simulink model "ekf1"  (R2023b)
settings: Solver=FixedStepAuto  StartTime=0.0  StopTime=Tend_slk  FixedStep=Ts_slk  RelTol=1e-3
values from neighbouring files (symbols this model uses):
  IMU_w_b_bias = IMU_var_bias_matrix(:,2)    [ekf1_script.m]    (also in ekf2_script.m; ekf3_script.m)
  meas_pole = 15    [ekf1_script.m]    (also in ekf2_script.m = 3; ekf3_script.m)
  P0 = diag([P0_ph,P0_th,P0_ps,P0_bias_wp,P0_bias_wq,P0_bias_wr])    [ekf1_script.m]
  Q = diag([q_ph,q_th,q_ps,q_bias_w_b,q_bias_w_b,q_bias_w_b])    [ekf1_script.m]
  R = diag([r_th,r_th,r_ps])    [ekf1_script.m]
  Ts_EKF_integr = 0.001    [complementary_filter_script.m]    (also in ekf1_script.m = 0.0001; ekf2_script.m = 0.0001; ekf3_script.m = 0.0001)
  Ts_EKF_meas = 0.01    [complementary_filter_script.m]    (also in ekf1_script.m; ekf2_script.m; ekf3_script.m)
  Ts_slk = 0.01    [complementary_filter_script.m]    (also in ekf1_script.m; ekf2_script.m; ekf3_script.m)
  x0EKF = [ph0;th0;ps0;bias_wp0;bias_wq0;bias_wr0]    [ekf1_script.m]
settings Model: Creator=teoma  LastModifiedBy=teoma

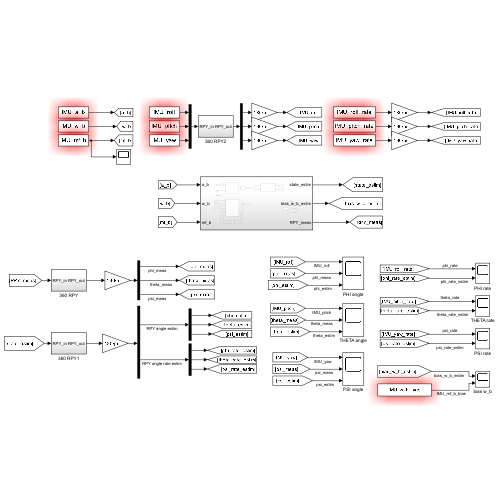
[thumbnail: Simulink's stored preview of the top-level diagram]
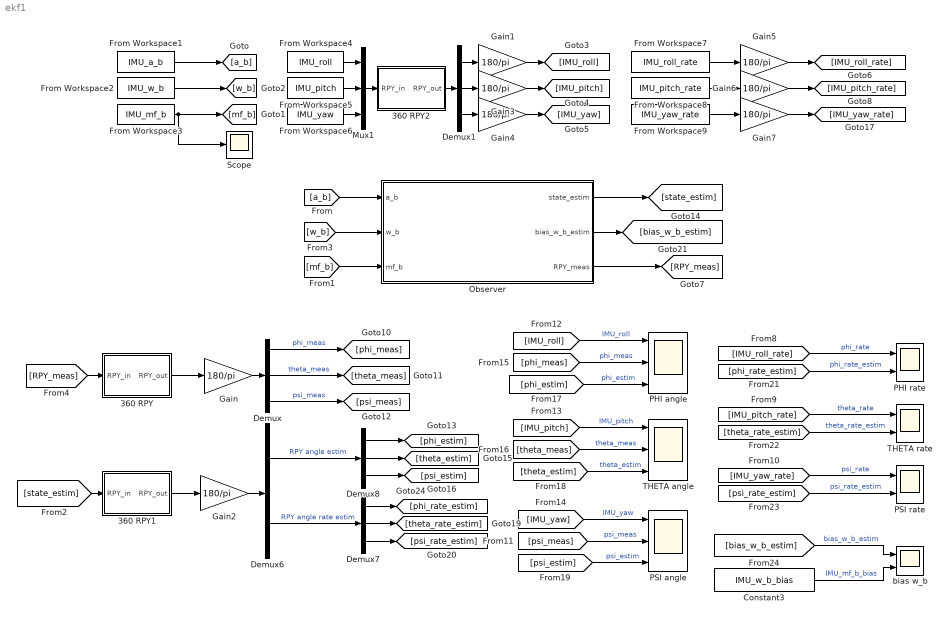
== system ekf1 ==
  360 RPY : Subsystem
  360 RPY1 : Subsystem
  360 RPY2 : Subsystem
  Constant3 : Constant  Value=IMU_w_b_bias
  Demux{,1,7..8} (4 alike) : Demux  Outputs=3
  Demux6 : Demux  Outputs=2
  From Workspace1 : FromWorkspace  VariableName=IMU_a_b  OutDataTypeStr=double  SampleTime=Ts_slk  Interpolate=off  OutputAfterFinalValue=Setting to zero
  From Workspace2 : FromWorkspace  VariableName=IMU_w_b  OutDataTypeStr=double  SampleTime=Ts_slk  Interpolate=off  OutputAfterFinalValue=Setting to zero
  From Workspace3 : FromWorkspace  VariableName=IMU_mf_b  OutDataTypeStr=double  SampleTime=Ts_slk  Interpolate=off  OutputAfterFinalValue=Setting to zero
  From Workspace4 : FromWorkspace  VariableName=IMU_roll  OutDataTypeStr=double  SampleTime=Ts_slk  Interpolate=off  OutputAfterFinalValue=Setting to zero
  From Workspace5 : FromWorkspace  VariableName=IMU_pitch  OutDataTypeStr=double  SampleTime=Ts_slk  Interpolate=off  OutputAfterFinalValue=Setting to zero
  From Workspace6 : FromWorkspace  VariableName=IMU_yaw  OutDataTypeStr=double  SampleTime=Ts_slk  Interpolate=off  OutputAfterFinalValue=Setting to zero
  From Workspace7 : FromWorkspace  VariableName=IMU_roll_rate  OutDataTypeStr=double  SampleTime=Ts_slk  Interpolate=off  OutputAfterFinalValue=Setting to zero
  From Workspace8 : FromWorkspace  VariableName=IMU_pitch_rate  OutDataTypeStr=double  SampleTime=Ts_slk  Interpolate=off  OutputAfterFinalValue=Setting to zero
  From Workspace9 : FromWorkspace  VariableName=IMU_yaw_rate  OutDataTypeStr=double  SampleTime=Ts_slk  Interpolate=off  OutputAfterFinalValue=Setting to zero
  Gain{,1..7} (8 alike) : Gain  Gain=180/pi
  Mux1 : Mux  Inputs=3
  Observer : Subsystem
  PHI angle : Scope  NumInputPorts=3
  PHI rate : Scope  NumInputPorts=2
  PSI angle : Scope  NumInputPorts=3
  PSI rate : Scope  NumInputPorts=2
  Scope : Scope
  THETA angle : Scope  NumInputPorts=3
  THETA rate : Scope  NumInputPorts=2
  bias w_b : Scope  NumInputPorts=2
  wires:
  Constant3/1 -> bias w_b/2  "IMU_mf_b_bias"
  [bias_w_b_estim] -> bias w_b/1  "bias_w_b_estim"
  [IMU_yaw_rate] -> PSI rate/1  "psi_rate"
  [theta_estim] -> THETA angle/3  "theta_estim"
  [theta_rate_estim] -> THETA rate/2  "theta_rate_estim"
  [IMU_pitch_rate] -> THETA rate/1  "theta_rate"
  [IMU_roll_rate] -> PHI rate/1  "phi_rate"
  [phi_rate_estim] -> PHI rate/2  "phi_rate_estim"
  [phi_estim] -> PHI angle/3  "phi_estim"
  [psi_estim] -> PSI angle/3  "psi_estim"
  [theta_meas] -> THETA angle/2  "theta_meas"
  [IMU_yaw] -> PSI angle/1  "IMU_yaw"
  [phi_meas] -> PHI angle/2  "phi_meas"
  [IMU_pitch] -> THETA angle/1  "IMU_pitch"
  [psi_rate_estim] -> PSI rate/2  "psi_rate_estim"
  [psi_meas] -> PSI angle/2  "psi_meas"
  [IMU_roll] -> PHI angle/1  "IMU_roll"
  From Workspace1/1 -> [a_b]
  From Workspace2/1 -> [w_b]
  From Workspace9/1 -> Gain7/1
  From Workspace8/1 -> Gain6/1
  From Workspace7/1 -> Gain5/1
  Gain5/1 -> [IMU_roll_rate]
  Gain6/1 -> [IMU_pitch_rate]
  Gain7/1 -> [IMU_yaw_rate]
  From Workspace3/1 -> [mf_b], Scope/1
  [mf_b] -> Observer/3(mf_b)
  [a_b] -> Observer/1(a_b)
  Observer/1(state_estim) -> [state_estim]
  Observer/2(bias_w_b_estim) -> [bias_w_b_estim]
  Observer/3(RPY_meas) -> [RPY_meas]
  [w_b] -> Observer/2(w_b)
  Demux8/2 -> [theta_estim]
  Demux8/3 -> [psi_estim]
  Demux7/3 -> [psi_rate_estim]
  Demux/2 -> [theta_meas]  "theta_meas"
  Gain/1 -> Demux/1
  Demux6/2 -> Demux7/1  "RPY angle rate estim"
  Demux7/2 -> [theta_rate_estim]
  360 RPY1/1(RPY_out) -> Gain2/1
  Demux6/1 -> Demux8/1  "RPY angle estim"
  360 RPY/1(RPY_out) -> Gain/1
  Demux8/1 -> [phi_estim]
  Demux7/1 -> [phi_rate_estim]
  Demux/3 -> [psi_meas]  "psi_meas"
  Gain2/1 -> Demux6/1
  Demux/1 -> [phi_meas]  "phi_meas"
  [state_estim] -> 360 RPY1/1(RPY_in)
  [RPY_meas] -> 360 RPY/1(RPY_in)
  Mux1/1 -> 360 RPY2/1(RPY_in)
  Demux1/1 -> Gain1/1
  From Workspace4/1 -> Mux1/1
  Gain1/1 -> [IMU_roll]
  Gain3/1 -> [IMU_pitch]
  Demux1/2 -> Gain3/1
  Demux1/3 -> Gain4/1
  From Workspace5/1 -> Mux1/2
  Gain4/1 -> [IMU_yaw]
  From Workspace6/1 -> Mux1/3
  360 RPY2/1(RPY_out) -> Demux1/1

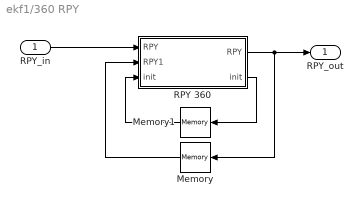
== system ekf1/360 RPY ==
  RPY_in : Inport
  Memory : Memory
  Memory1 : Memory
  RPY 360 : MATLAB Function  TreatAsAtomicUnit=on
  RPY_out : Outport
  wires:
  Memory/1 -> RPY 360/2(RPY1)
  Memory1/1 -> RPY 360/3("init ")
  RPY 360/2(init) -> Memory1/1
  RPY 360/1(RPY) -> Memory/1, RPY_out/1
  RPY_in/1 -> RPY 360/1("RPY ")

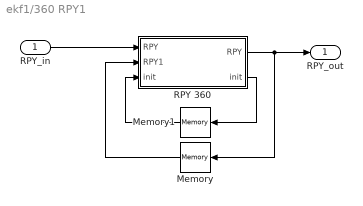
== system ekf1/360 RPY1 ==
  RPY_in : Inport
  Memory : Memory
  Memory1 : Memory
  RPY 360 : MATLAB Function  TreatAsAtomicUnit=on
  RPY_out : Outport
  wires:
  Memory/1 -> RPY 360/2(RPY1)
  Memory1/1 -> RPY 360/3("init ")
  RPY 360/2(init) -> Memory1/1
  RPY 360/1(RPY) -> Memory/1, RPY_out/1
  RPY_in/1 -> RPY 360/1("RPY ")

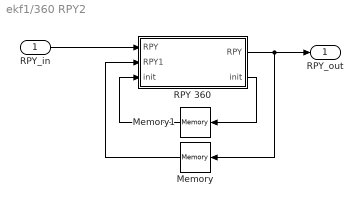
== system ekf1/360 RPY2 ==
  RPY_in : Inport
  Memory : Memory
  Memory1 : Memory
  RPY 360 : MATLAB Function  TreatAsAtomicUnit=on
  RPY_out : Outport
  wires:
  RPY_in/1 -> RPY 360/1("RPY ")
  RPY 360/1(RPY) -> Memory/1, RPY_out/1
  Memory/1 -> RPY 360/2(RPY1)
  RPY 360/2(init) -> Memory1/1
  Memory1/1 -> RPY 360/3("init ")

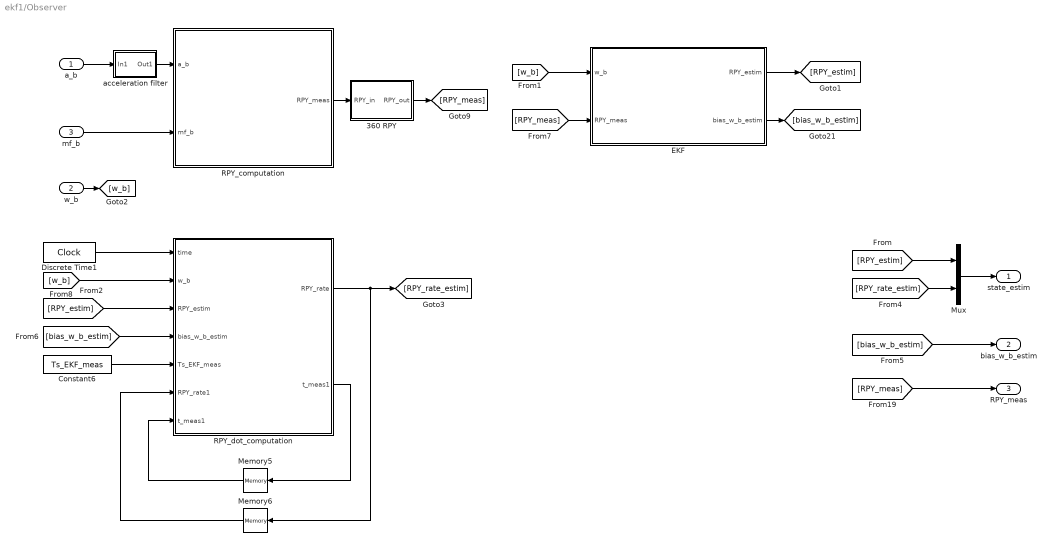
== system ekf1/Observer ==
  a_b : Inport
  w_b : Inport  Port=2
  mf_b : Inport  Port=3
  360 RPY : Subsystem
  Constant6 : Constant  Value=Ts_EKF_meas
  Discrete Time1 : DigitalClock  SampleTime=Ts_slk
  EKF : Subsystem
  Memory5 : Memory
  Memory6 : Memory
  Mux : Mux  Inputs=2
  RPY_computation : MATLAB Function  TreatAsAtomicUnit=on
  RPY_dot_computation : MATLAB Function  TreatAsAtomicUnit=on
  acceleration filter : Subsystem  mask{p=meas_pole}
      mask prompts: p "pole (p)"
  state_estim : Outport
  bias_w_b_estim : Outport  Port=2
  RPY_meas : Outport  Port=3
  wires:
  [w_b] -> EKF/1(w_b)
  EKF/1(RPY_estim) -> [RPY_estim]
  a_b/1 -> acceleration filter/1(In1)
  acceleration filter/1(Out1) -> RPY_computation/1(a_b)
  [RPY_meas] -> EKF/2(RPY_meas)
  EKF/2(bias_w_b_estim) -> [bias_w_b_estim]
  RPY_computation/1(RPY_meas) -> 360 RPY/1(RPY_in)
  mf_b/1 -> RPY_computation/2(mf_b)
  Memory5/1 -> RPY_dot_computation/7("t_meas1 ")
  Discrete Time1/1 -> RPY_dot_computation/1(time)
  RPY_dot_computation/2(t_meas1) -> Memory5/1
  [w_b] -> RPY_dot_computation/2(w_b)
  Memory6/1 -> RPY_dot_computation/6(RPY_rate1)
  RPY_dot_computation/1(RPY_rate) -> [RPY_rate_estim], Memory6/1
  Constant6/1 -> RPY_dot_computation/5(Ts_EKF_meas)
  [RPY_estim] -> RPY_dot_computation/3(RPY_estim)
  [bias_w_b_estim] -> RPY_dot_computation/4(bias_w_b_estim)
  w_b/1 -> [w_b]
  [RPY_meas] -> RPY_meas/1
  [bias_w_b_estim] -> bias_w_b_estim/1
  Mux/1 -> state_estim/1
  [RPY_estim] -> Mux/1
  [RPY_rate_estim] -> Mux/2
  360 RPY/1(RPY_out) -> [RPY_meas]

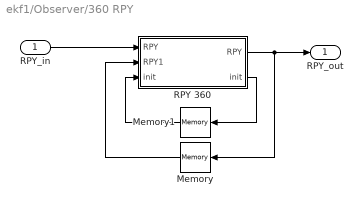
== system ekf1/Observer/360 RPY ==
  RPY_in : Inport
  Memory : Memory
  Memory1 : Memory
  RPY 360 : MATLAB Function  TreatAsAtomicUnit=on
  RPY_out : Outport
  wires:
  RPY_in/1 -> RPY 360/1("RPY ")
  RPY 360/1(RPY) -> Memory/1, RPY_out/1
  Memory/1 -> RPY 360/2(RPY1)
  RPY 360/2(init) -> Memory1/1
  Memory1/1 -> RPY 360/3("init ")

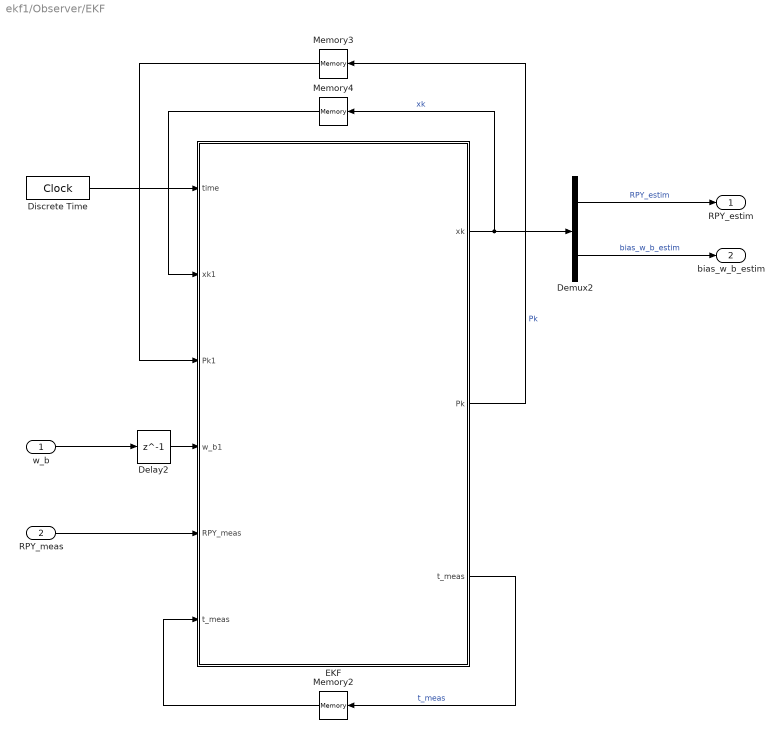
== system ekf1/Observer/EKF ==
  w_b : Inport
  RPY_meas : Inport  Port=2
  Delay2 : Delay  DelayLength=1  SampleTime=Ts_EKF_meas
  Demux2 : Demux  Outputs=2
  Discrete Time : DigitalClock  SampleTime=Ts_slk
  EKF : MATLAB Function  TreatAsAtomicUnit=on
  Memory2 : Memory
  Memory3 : Memory  InitialCondition=P0
  Memory4 : Memory  InitialCondition=x0EKF
  RPY_estim : Outport
  bias_w_b_estim : Outport  Port=2
  wires:
  w_b/1 -> Delay2/1
  EKF/2(Pk) -> Memory3/1  "Pk"
  Memory2/1 -> EKF/6("t_meas ")
  EKF/3(t_meas) -> Memory2/1  "t_meas"
  RPY_meas/1 -> EKF/5(RPY_meas)
  Discrete Time/1 -> EKF/1(time)
  Memory3/1 -> EKF/3(Pk1)
  Delay2/1 -> EKF/4(w_b1)
  Memory4/1 -> EKF/2(xk1)
  Demux2/2 -> bias_w_b_estim/1  "bias_w_b_estim"
  EKF/1(xk) -> Memory4/1, Demux2/1  "xk"
  Demux2/1 -> RPY_estim/1  "RPY_estim"

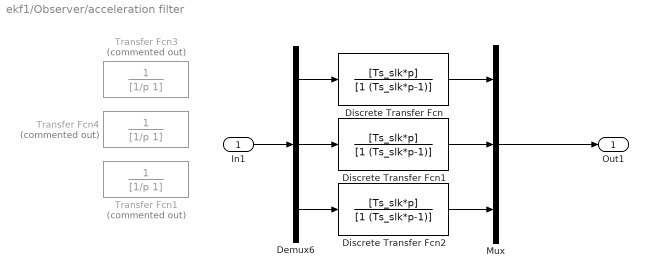
== system ekf1/Observer/acceleration filter ==
  In1 : Inport
  Demux6 : Demux  Outputs=3
  Discrete Transfer Fcn : DiscreteTransferFcn  Numerator=[Ts_slk*p]  Denominator=[1 (Ts_slk*p-1)]
  Discrete Transfer Fcn1 : DiscreteTransferFcn  Numerator=[Ts_slk*p]  Denominator=[1 (Ts_slk*p-1)]
  Discrete Transfer Fcn2 : DiscreteTransferFcn  Numerator=[Ts_slk*p]  Denominator=[1 (Ts_slk*p-1)]
  Mux : Mux  Inputs=3
  Transfer Fcn1 : TransferFcn  Commented=on  Denominator=[1/p 1]
  Transfer Fcn3 : TransferFcn  Commented=on  Denominator=[1/p 1]
  Transfer Fcn4 : TransferFcn  Commented=on  Denominator=[1/p 1]
  Out1 : Outport
  wires:
  Discrete Transfer Fcn1/1 -> Mux/2
  Demux6/3 -> Discrete Transfer Fcn2/1
  Mux/1 -> Out1/1
  Discrete Transfer Fcn2/1 -> Mux/3
  Discrete Transfer Fcn/1 -> Mux/1
  In1/1 -> Demux6/1
  Demux6/1 -> Discrete Transfer Fcn/1
  Demux6/2 -> Discrete Transfer Fcn1/1

== matlab function ekf1/Observer/RPY_dot_computation ==
  data: time input; w_b input; RPY_estim input; bias_w_b_estim input; Ts_EKF_meas input; RPY_rate1 input; RPY_rate output; t_meas1 input; t_meas1 output
function [RPY_rate,t_meas1] = RPY_dot_computation(time,w_b,RPY_estim,bias_w_b_estim,Ts_EKF_meas,RPY_rate1,t_meas1)

if time - t_meas1 >= Ts_EKF_meas || time == 0
    wp          =       w_b(1,1);               % p-dir of angular velocity w
    wq          =       w_b(2,1);               % q-dir of angular velocity w
    wr          =       w_b(3,1);               % r-dir of angular velocity w

    phi         =       RPY_estim(1,1);         % roll angle (rad)
    theta       =       RPY_estim(2,1);         % pitch angle (rad)
    psi         =       RPY_estim(3,1);         % yaw angle (rad)  
    bias_wp     =       bias_w_b_estim(1,1);    % bias of p-dir of angular velocity w
    bias_wq     =       bias_w_b_estim(2,1);    % bias of q-dir of angular velocity w
    bias_wr     =       bias_w_b_estim(3,1);   % bias of r-dir of angular velocity w

    cph         =       cos(phi);
    cth         =       cos(theta);
    cps         =       cos(psi);
    sph         =       sin(phi);
    sth         =       sin(theta);
    sps         =       sin(psi);
    tth         =       sth/cth;

    % integration step
    t_meas1 = time;
    W_eta = [1,    sph*tth,    cph*tth;
             0,    cph,        -sph;
             0,    sph/cth,    cph/cth;];
    w_b_corrected = [wp-bias_wp; wq-bias_wq; wr-bias_wr;];
    RPY_rate = W_eta*w_b_corrected;
else
    RPY_rate = RPY_rate1;
end
end

== matlab function ekf1/360 RPY1/RPY 360 ==
  data: RPY input; RPY output; RPY1 input; init output; init input
function [RPY,init] = RPY_360(RPY,RPY1,init)
if init < 2 
    if init == 0
        init = 1;
        RPY1 = RPY;
    elseif init == 1
        if (RPY - RPY1)'*(RPY - RPY1) > 0.01
            init = 2;
            RPY1 = RPY;
        end
    end
end

% - pi <= PHI <= + pi PHI uses atan2()
if abs(RPY(1) - RPY1(1)) > pi*0.99
    RPY(1) = RPY(1) + sign(RPY1(1))*(2*pi);
end
% - pi/2 <= THETA <= + pi/2 THETA uses asin()
if abs(RPY(2) - RPY1(2)) > pi/2*0.99
    RPY(2) = RPY(2) + sign(RPY1(2))*(2*pi);
end
% - pi <= PSI <= + pi PSI uses atan2()
if abs(RPY(3) - RPY1(3)) > pi*0.99
    RPY(3) = RPY(3) + sign(RPY1(3))*(2*pi);
end
end

== matlab function ekf1/Observer/360 RPY/RPY 360 ==
  data: RPY input; RPY output; RPY1 input; init output; init input
function [RPY,init] = RPY_360(RPY,RPY1,init)
if init < 2 
    if init == 0
        init = 1;
        RPY1 = RPY;
    elseif init == 1
        if (RPY - RPY1)'*(RPY - RPY1) > 0.01
            init = 2;
            RPY1 = RPY;
        end
    end
end

% - pi <= PHI <= + pi PHI uses atan2()
if abs(RPY(1) - RPY1(1)) > pi*0.99
    RPY(1) = RPY(1) + sign(RPY1(1))*(2*pi);
end
% - pi/2 <= THETA <= + pi/2 THETA uses asin()
if abs(RPY(2) - RPY1(2)) > pi/2*0.99
    RPY(2) = RPY(2) + sign(RPY1(2))*(2*pi);
end
% - pi <= PSI <= + pi PSI uses atan2()
if abs(RPY(3) - RPY1(3)) > pi*0.99
    RPY(3) = RPY(3) + sign(RPY1(3))*(2*pi);
end
end

== matlab function ekf1/Observer/RPY_computation ==
  data: a_b input; mf_b input; RPY_meas output
function RPY_meas    = RPY_computation(a_b,mf_b)
% description:
% - a_b             = measured linear acceleration in body-frame
% - w_b             = measured angular velocity in body-frame
% - mf_b            = measured magnetic field in body-frame
% - mf              = measured magnetic field in body-inertia
% - a_b_disturbe    = linear velocity measurement-noise
% - w_b_disturbe    = angular velocity measurement-noise
% - mf_b_disturbe   = magnetic field measurement-noise

% -------------------------------------------------------------------------------------------
% observation: the following computation works only if the angles
% phi,theta,psy are withing angles (-pi/2,+pi/2) (this is an open set, pi/2 is excluded)
% -------------------------------------------------------------------------------------------

a_b = -1*a_b;       % need to adjust the sign to use atan2() function correctly

% phi computation
ph_meas = atan2(a_b(2), a_b(3));
sph = sin(ph_meas);
cph = cos(ph_meas);

% theta computation
th_meas = atan2(-a_b(1), (a_b(2)*sph + a_b(3)*cph));
sth = sin(th_meas);
cth = cos(th_meas);

% psi computation
ps_meas_num   = mf_b(3)*sph - mf_b(2)*cph;
ps_meas_den   = mf_b(1)*cth + mf_b(2)*sth*sph + mf_b(3)*sth*cph;
ps_meas = atan2(ps_meas_num, ps_meas_den);

RPY_meas = [ph_meas;th_meas;ps_meas];

== matlab function ekf1/Observer/EKF/EKF ==
  data: time input; xk1 input; Pk1 input; w_b1 input; RPY_meas input; t_meas input; Q parameter; xk output; Pk output; t_meas output; R parameter; Ts_EKF_integr parameter; Ts_EKF_meas parameter
function [xk,Pk,t_meas] = EKF(time,xk1,Pk1,w_b1,RPY_meas,t_meas,Q,R,Ts_EKF_integr,Ts_EKF_meas)

if time - t_meas >= Ts_EKF_meas
    t_meas = time;

  % INTEGRATION STEP
    % initial condition
    xt1         =       xk1;                        % initial condition for the state
    Pt1         =       Pk1;                        % initial condition for matrix P

    wp1         =       w_b1(1,1);                  % past value of the p-dir of angular velocity w
    wq1         =       w_b1(2,1);                  % past value of the q-dir of angular velocity w
    wr1         =       w_b1(3,1);                  % past value of the r-dir of angular velocity w
    % integration loop
    Nstep       = floor(Ts_EKF_meas/Ts_EKF_integr); % number of integration steps to performe in the t_meas time windows
    xt          = zeros(6,1);
    Pt          = zeros(6,6);
    for i = 1:1:Nstep
        % state extraction
            phi         =       xt1(1,1);           % roll angle (rad)
            theta       =       xt1(2,1);           % pitch angle (rad)
            psi         =       xt1(3,1);           % yaw angle (rad)  
            bias_wp     =       xt1(4,1);           % bias of p-dir of angular velocity w
            bias_wq     =       xt1(5,1);           % bias of q-dir of angular velocity w
            bias_wr     =       xt1(6,1);           % bias of r-dir of angular velocity w
        
            cph         =       cos(phi);
            cth         =       cos(theta);
            cps         =       cos(psi);
            sph         =       sin(phi);
            sth         =       sin(theta);
            sps         =       sin(psi);
            tth         =       sth/cth;
        % integration
            Mf = [1,    sph*tth,    cph*tth,    0,  0,  0;
                  0,    cph,        -sph,       0,  0,  0;
                  0,    sph/cth,    cph/cth,    0,  0,  0;
                  0,    0,          0,          0,  0,  0;
                  0,    0,          0,          0,  0,  0;
                  0,    0,          0,          0,  0,  0;];
            Z1 = [wp1-bias_wp; wq1-bias_wq; wr1-bias_wr; bias_wp; bias_wq; bias_wr;];
            f = Mf*Z1;
            xt = xt1 + Ts_EKF_integr*f;
        
            A1 = [cph*tth*(wq1-bias_wq)-sph*tth*(wr1-bias_wr),(sph*(wq1-bias_wq)+cph*(wr1-bias_wr))/cth^2,  0,  -1, -sph*tth,   -cph*tth;];
            A2 = [-sph*(wq1-bias_wq)-cph*(wr1-bias_wr),   0,  0,  0,  -cph,   sph;];
            A3 = [0,  0,  0,  0,  0,  0;];
            A4 = [0,  0,  0,  0,  0,  0;];
            A5 = [0,  0,  0,  0,  0,  0;];
            A6 = [0,  0,  0,  0,  0,  0;];
            At1 = [A1; A2; A3; A4; A5; A6;];
            Pt = Pt1 + Ts_EKF_integr*(At1*Pt1 + Pt1*At1' + Q);
        % house keeping
            xt1 = xt;
            Pt1 = Pt;
    end
  % MEASUREMENT STEP
    Ck = [eye(3),zeros(3,3)];
    Lk = Pt*Ck'/(Ck*Pt*Ck' + R);
    xk = xt + Lk*(RPY_meas - Ck*xt);
    Pk = (eye(6) - Lk*Ck)*Pt;
else
    xk = xk1;
    Pk = Pk1;
end
end

== matlab function ekf1/360 RPY/RPY 360 ==
  data: RPY input; RPY output; RPY1 input; init output; init input
function [RPY,init] = RPY_360(RPY,RPY1,init)
if init < 2 
    if init == 0
        init = 1;
        RPY1 = RPY;
    elseif init == 1
        if (RPY - RPY1)'*(RPY - RPY1) > 0.01
            init = 2;
            RPY1 = RPY;
        end
    end
end

% - pi <= PHI <= + pi PHI uses atan2()
if abs(RPY(1) - RPY1(1)) > pi*0.99
    RPY(1) = RPY(1) + sign(RPY1(1))*(2*pi);
end
% - pi/2 <= THETA <= + pi/2 THETA uses asin()
if abs(RPY(2) - RPY1(2)) > pi/2*0.99
    RPY(2) = RPY(2) + sign(RPY1(2))*(2*pi);
end
% - pi <= PSI <= + pi PSI uses atan2()
if abs(RPY(3) - RPY1(3)) > pi*0.99
    RPY(3) = RPY(3) + sign(RPY1(3))*(2*pi);
end
end

== matlab function ekf1/360 RPY2/RPY 360 ==
  data: RPY input; RPY output; RPY1 input; init output; init input
function [RPY,init] = RPY_360(RPY,RPY1, init)
if init < 2 
    if init == 0
        init = 1;
        RPY1 = RPY;
    elseif init == 1
        if (RPY - RPY1)'*(RPY - RPY1) > 0.01
            init = 2;
        else
            RPY1 = RPY;
        end
    end
end

% - pi <= PHI <= + pi PHI uses atan2()
if abs(RPY(1) - RPY1(1)) > pi/2
    RPY(1) = RPY(1) + sign(RPY1(1))*(2*pi);
end
% - pi/2 <= THETA <= + pi/2 THETA uses asin()
if abs(RPY(2) - RPY1(2)) > pi/2
    RPY(2) = RPY(2) + sign(RPY1(2))*(2*pi);
end
% - pi <= PSI <= + pi PSI uses atan2()
if abs(RPY(3) - RPY1(3)) > pi/2
    RPY(3) = RPY(3) + sign(RPY1(3))*(2*pi);
end
end
